simulink model "part4"  (R2024a)
settings: Solver=VariableStepAuto  StartTime=0.0  StopTime=50  RelTol=1e-3
undefined symbols (not defined in the file or in its folder): magnitude
settings Model: Creator=katutu  LastModifiedBy=katutu

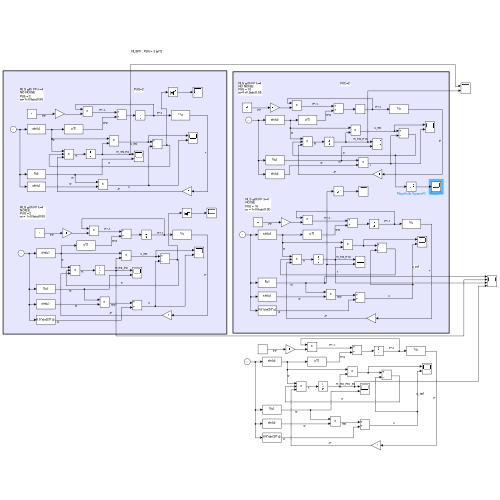
[thumbnail: Simulink's stored preview of the top-level diagram]
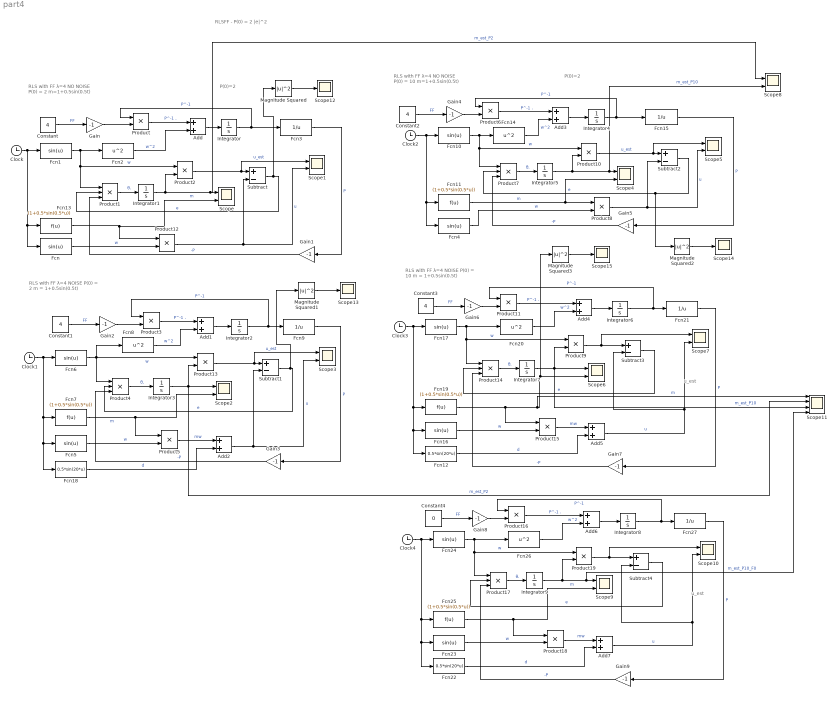
== system part4 ==
  note: RLSFF - P(0) = 2 |e|^2
  note: RLS with FF λ=4
      | NO NOISE
      | P(0) = 2
      | m=1+0.5sin(0.5t)
  note: P(0)=2
  note: RLS with FF λ=4
      | NOISE
      | P(0) = 2
      | m = 1+0.5sin(0.5t)
  note: RLS with FF λ=4
      | NOISE
      | P(0) = 10
      | m = 1+0.5sin(0.5t)
  note: RLS with FF λ=4
      | NO NOISE
      | P(0) = 10
      | m=1+0.5sin(0.5t)
  note: P(0)=2
  note: u_est
  note: u_est
  Add{,1..7} (8 alike) : Sum
  Clock{,1..4} (5 alike) : Clock
  Constant{,1..3} (4 alike) : Constant  Value=4
  Constant4 : Constant  Value=0
  Fcn{,1,4..6,10,16..17,23..24} (10 alike) : Fcn  Expr=sin(u)
  Fcn{7,11,13,19,25} (5 alike) : Fcn  Expr=(1+0.5*sin(0.5*u))
  Fcn12 : Fcn  Expr=0.5*sin(20*u)
  Fcn{2,8,14,20,26} (5 alike) : Fcn  Expr=u^2
  Fcn{3,9,15,21,27} (5 alike) : Fcn  Expr=1/u
  Fcn18 : Fcn  Expr=0.5*sin(20*u)
  Fcn22 : Fcn  Expr=0.5*sin(20*u)
  Gain{,1..9} (10 alike) : Gain  Gain=-1
  Integrator{,1..3,5,7,9} (7 alike) : Integrator  InitialCondition=0.5
  Integrator4 : Integrator  InitialCondition=0.1
  Integrator6 : Integrator  InitialCondition=0.1
  Integrator8 : Integrator  InitialCondition=0.1
  Magnitude Squared{,1..3} (4 alike) : Math  Operator=magnitude^2
  Product{,2..3,5..6,8..13,15..16,18..19} (15 alike) : Product
  Product{1,4,7,14,17} (5 alike) : Product  Inputs=3
  Scope{,1..10} (11 alike) : Scope  NumInputPorts=2
  Scope11 : Scope  NumInputPorts=4
  Scope{12..15} (4 alike) : Scope
  Subtract{,1..4} (5 alike) : Sum  Inputs=+-
  wires:
  Integrator/1 -> Product/1, Fcn3/1  "P^-1"
  Fcn3/1 -> Gain1/1  "P"
  Subtract/1 -> Magnitude Squared/1, Product1/2  "e"
  Product/1 -> Add/1  "P^-1 ."
  Product1/1 -> Integrator1/1  "θ."
  Fcn1/1 -> Product1/1, Product2/1, Fcn2/1  "w"
  Product2/1 -> Scope1/1, Subtract/1  "u_est"
  Constant/1 -> Gain/1  "FF"
  Gain/1 -> Product/2
  Add/1 -> Integrator/1
  Integrator1/1 -> Scope8/1, Scope/1, Product2/2  "m_est_P2"
  Clock/1 -> Fcn/1, Fcn13/1, Fcn1/1
  Fcn2/1 -> Add/2  "w^2"
  Gain1/1 -> Product1/3  "-P"
  Fcn13/1 -> Product12/1, Scope/2  "m"
  Fcn/1 -> Product12/2  "w"
  Product12/1 -> Scope1/2, Subtract/2  "u"
  Product13/1 -> Subtract1/1, Scope3/1  "u_est"
  Integrator3/1 -> Scope11/2, Product13/2, Scope2/1  "m_est_P2"
  Fcn9/1 -> Gain3/1  "P"
  Clock1/1 -> Fcn6/1, Fcn18/1, Fcn5/1, Fcn7/1
  Constant1/1 -> Gain2/1  "FF"
  Gain3/1 -> Product4/3  "-P"
  Integrator2/1 -> Product3/1, Fcn9/1  "P^-1"
  Product4/1 -> Integrator3/1  "θ."
  Add1/1 -> Integrator2/1
  Fcn6/1 -> Fcn8/1, Product13/1, Product4/1  "w"
  Fcn8/1 -> Add1/2  "w^2"
  Subtract1/1 -> Magnitude Squared1/1, Product4/2  "e"
  Product3/1 -> Add1/1  "P^-1 ."
  Fcn7/1 -> Product5/1, Scope2/2  "m"
  Gain2/1 -> Product3/2
  Add2/1 -> Scope3/2, Subtract1/2  "u"
  Fcn5/1 -> Product5/2  "w"
  Product5/1 -> Add2/1  "mw"
  Fcn18/1 -> Add2/2  "d"
  Product10/1 -> Scope5/1, Subtract2/1  "u_est"
  Integrator5/1 -> Scope8/2, Scope4/1, Product10/2  "m_est_P10"
  Product15/1 -> Add5/1  "mw"
  Clock2/1 -> Fcn4/1, Fcn11/1, Fcn10/1
  Subtract3/1 -> Product14/2  "e"
  Constant2/1 -> Gain4/1  "FF"
  Integrator6/1 -> Fcn21/1, Product11/1  "P^-1"
  Subtract2/1 -> Magnitude Squared2/1, Product7/2  "e"
  Product7/1 -> Integrator5/1  "θ."
  Fcn10/1 -> Product7/1, Product10/1, Fcn14/1  "w"
  Fcn15/1 -> Gain5/1  "P"
  Gain6/1 -> Product11/2
  Gain5/1 -> Product7/3  "-P"
  Product11/1 -> Add4/1  "P^-1 ."
  Add4/1 -> Integrator6/1
  Fcn19/1 -> Product15/1, Scope11/1, Magnitude Squared3/1, Scope6/2  "m"
  Product14/1 -> Integrator7/1  "θ."
  Fcn20/1 -> Add4/2  "w^2"
  Fcn17/1 -> Product14/1, Product9/1, Fcn20/1  "w"
  Integrator4/1 -> Fcn15/1, Product6/1  "P^-1"
  Add3/1 -> Integrator4/1
  Fcn14/1 -> Add3/2  "w^2"
  Gain7/1 -> Product14/3  "-P"
  Product6/1 -> Add3/1  "P^-1 ."
  Fcn11/1 -> Scope4/2, Product8/1  "m"
  Fcn16/1 -> Product15/2  "w"
  Add5/1 -> Scope7/2, Subtract3/2  "u"
  Fcn12/1 -> Add5/2  "d"
  Fcn4/1 -> Product8/2  "w"
  Gain4/1 -> Product6/2
  Product8/1 -> Scope5/2, Subtract2/2  "u"
  Constant3/1 -> Gain6/1  "FF"
  Integrator7/1 -> Scope11/3, Scope6/1, Product9/2  "m_est_P10"
  Product9/1 -> Subtract3/1, Scope7/1
  Fcn21/1 -> Gain7/1  "P"
  Clock3/1 -> Fcn12/1, Fcn16/1, Fcn19/1, Fcn17/1
  Constant4/1 -> Gain8/1  "FF"
  Integrator9/1 -> Scope11/4, Scope9/1, Product19/2  "m_est_P10_F0"
  Subtract4/1 -> Product17/2  "e"
  Product16/1 -> Add6/1  "P^-1 ."
  Fcn27/1 -> Gain9/1  "P"
  Integrator8/1 -> Fcn27/1, Product16/1  "P^-1"
  Product19/1 -> Subtract4/1, Scope10/1
  Add7/1 -> Scope10/2, Subtract4/2  "u"
  Product18/1 -> Add7/1  "mw"
  Fcn25/1 -> Product18/1, Scope9/2  "m"
  Gain8/1 -> Product16/2
  Fcn22/1 -> Add7/2  "d"
  Fcn23/1 -> Product18/2  "w"
  Product17/1 -> Integrator9/1  "θ."
  Add6/1 -> Integrator8/1
  Fcn24/1 -> Product17/1, Product19/1, Fcn26/1  "w"
  Gain9/1 -> Product17/3  "-P"
  Fcn26/1 -> Add6/2  "w^2"
  Clock4/1 -> Fcn22/1, Fcn23/1, Fcn25/1, Fcn24/1
  Magnitude Squared/1 -> Scope12/1
  Magnitude Squared1/1 -> Scope13/1
  Magnitude Squared2/1 -> Scope14/1
  Magnitude Squared3/1 -> Scope15/1
